simulink model "circuito_RLC_modelo"  (R2020b)
settings: Solver=VariableStepAuto  StartTime=0.0  StopTime=1.5  RelTol=1e-3
values from neighbouring files (symbols this model uses):
  C = [0 1 0 0 0;0 0 0 1 0]    [modelo.m]    (also in simu_RLC_modelo.m = 2e-05)
  E = 2*alpha.*sin(2*pi*fs.*(v.*t./c+(d-dr)/c)).*sin(2*pi*fs.*(t-d/c))    [literal_a.m]    (also in simu_RLC_modelo.m = 12)
  L = linspace(0.1e-3,0.51e-3,10)    [modelo.m]    (also in simu_RLC_modelo.m = 0.1)
  R = 30455.3    [modelo.m]    (also in simu_RLC_modelo.m = 100)
settings Model: Creator=Mateo  LastModifiedBy=Mateo
settings DataIOCC: ReturnWorkspaceOutputs=off

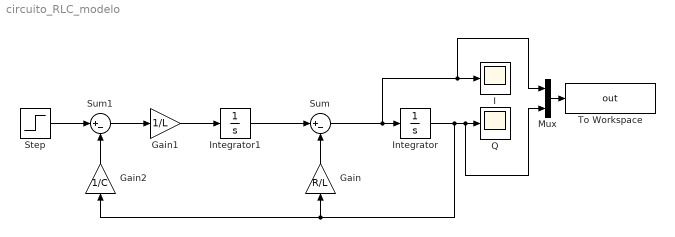
== system circuito_RLC_modelo ==
  Gain : Gain  Gain=R/L
  Gain1 : Gain  Gain=1/L
  Gain2 : Gain  Gain=1/C
  I : Scope
  Integrator : Integrator
  Integrator1 : Integrator
  Mux : Mux  Inputs=2
  Q : Scope
  Step : Step  After=E  SampleTime=0
  Sum : Sum  Inputs=|+-
  Sum1 : Sum  Inputs=|+-
  To Workspace : ToWorkspace  VariableName=out  SaveFormat=Timeseries  SampleTime=-1
  wires:
  Gain/1 -> Sum/2
  Sum/1 -> Mux/1, I/1, Integrator/1
  Gain1/1 -> Integrator1/1
  Integrator1/1 -> Sum/1
  Step/1 -> Sum1/1
  Sum1/1 -> Gain1/1
  Gain2/1 -> Sum1/2
  Integrator/1 -> Mux/2, Q/1, Gain/1, Gain2/1
  Mux/1 -> To Workspace/1
